simulink model "Model_SD_CIFB_k2_TC"  (Simulink 10.0)
settings: Solver=ode45  StartTime=0.0  StopTime=Tstop  RelTol=1e-3  EnableMultiTasking=on
values from neighbouring files (symbols this model uses):
  Amp = 10^(Av/20)*FS    (= 0.501187233627)    [run_Model_SD_CIFB_k2.m]
  fs = 2*BA*OSR    (= 2560000)    [run_Model_SD_CIFB_k2.m]
  OSR = 64    [run_Model_SD_CIFB_k2.m]
  ts = 1/fs    (= 3.90625e-07)    [run_Model_SD_CIFB_k2.m]
  win = 2*pi*fin    [run_Model_SD_CIFB_k2.m]
settings Model: LogicAnalyzerSignalOrdering=a7e547d9-241f-4ffb-821e-5a0431325834  Creator=cellierr  LastModifiedBy=corentin.pichat
settings DataIOCC: LimitDataPoints=on
settings OptimizationCC: ExpressionDepthLimit=2147483647  InitFltsAndDblsToZero=on
settings DebuggingCC: SaveWithParameterizedLinksMsg=none  SolverPrmCheckMsg=warning  FcnCallInpInsideContextMsg=warning  StateNameClashWarn=warning
settings GRTTargetCC: TargetFcnLib=ansi_tfl_tmw.mat  GeneratePreprocessorConditionals=Disable all
settings ConfigComp: CovExternalEMLEnable=off  CovSFcnEnable=off

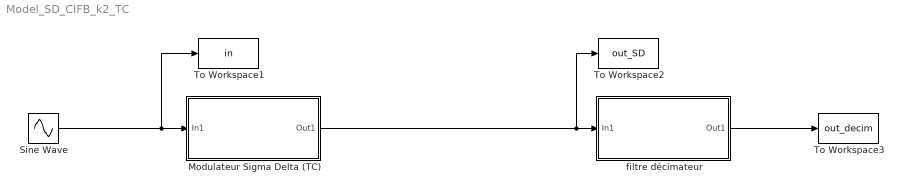
== system Model_SD_CIFB_k2_TC ==
  Modulateur Sigma Delta (TC) : Subsystem
  Sine Wave : Sin  Amplitude=Amp  Frequency=win  SampleTime=0
  To Workspace1 : ToWorkspace  VariableName=in  SampleTime=-1
  To Workspace2 : ToWorkspace  VariableName=out_SD  SampleTime=-1
  To Workspace3 : ToWorkspace  VariableName=out_decim  SampleTime=ts
  filtre décimateur : Subsystem
  wires:
  Sine Wave/1 -> To Workspace1/1, Modulateur Sigma Delta (TC)/1(In1)
  filtre décimateur/1(Out1) -> To Workspace3/1
  Modulateur Sigma Delta (TC)/1(Out1) -> filtre décimateur/1(In1), To Workspace2/1

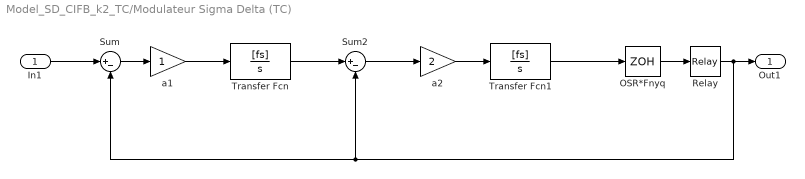
== system Model_SD_CIFB_k2_TC/Modulateur Sigma Delta (TC) ==
  In1 : Inport
  OSR*Fnyq : ZeroOrderHold  SampleTime=1/(fs)
  Relay : Relay  OnSwitchValue=0  OffSwitchValue=0  OffOutputValue=-1
  Sum : Sum  Inputs=|+-
  Sum2 : Sum  Inputs=|+-
  Transfer Fcn : TransferFcn  Numerator=[fs]  Denominator=[1 0]
  Transfer Fcn1 : TransferFcn  Numerator=[fs]  Denominator=[1 0]
  a1 : Gain
  a2 : Gain  Gain=2
  Out1 : Outport
  wires:
  In1/1 -> Sum/1
  Sum/1 -> a1/1
  Sum2/1 -> a2/1
  Relay/1 -> Sum2/2, Sum/2, Out1/1
  OSR*Fnyq/1 -> Relay/1
  a1/1 -> Transfer Fcn/1
  Transfer Fcn/1 -> Sum2/1
  a2/1 -> Transfer Fcn1/1
  Transfer Fcn1/1 -> OSR*Fnyq/1

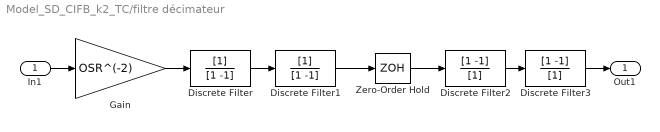
== system Model_SD_CIFB_k2_TC/filtre décimateur ==
  In1 : Inport
  Discrete Filter : DiscreteFilter  Denominator=[1 -1]
  Discrete Filter1 : DiscreteFilter  Denominator=[1 -1]
  Discrete Filter2 : DiscreteFilter  Numerator=[1 -1]  Denominator=[1]  SampleTime=ts*OSR
  Discrete Filter3 : DiscreteFilter  Numerator=[1 -1]  Denominator=[1]  SampleTime=ts*OSR
  Gain : Gain  Gain=OSR^(-2)  SaturateOnIntegerOverflow=on  OutDataTypeStr=Inherit: Same as input  ParamDataTypeStr=Inherit: Same as input
  Zero-Order Hold : ZeroOrderHold  SampleTime=ts*OSR
  Out1 : Outport
  wires:
  In1/1 -> Gain/1
  Discrete Filter3/1 -> Out1/1
  Gain/1 -> Discrete Filter/1
  Discrete Filter/1 -> Discrete Filter1/1
  Discrete Filter2/1 -> Discrete Filter3/1
  Discrete Filter1/1 -> Zero-Order Hold/1
  Zero-Order Hold/1 -> Discrete Filter2/1
